simulink model "MOTORfault"  (R2018a)
settings: Solver=ode23tb  StartTime=0.0  StopTime=5  RelTol=1e-3  EnableMultiTasking=on
libraries: powerlib x1
settings Model: Creator=MAY  LastModifiedBy=MAY
settings DataIOCC: LimitDataPoints=on  SaveFormat=Array  SignalLoggingSaveFormat=ModelDataLogs  SignalLoggingName=sigsOut
settings DebuggingCC: SaveWithParameterizedLinksMsg=none  UnderspecifiedInitializationDetection=Classic  MergeDetectMultiDrivingBlocksExec=none  SignalResolutionControl=TryResolveAllWithWarning  MultiTaskDSMMsg=warning  MultiTaskCondExecSysMsg=none
settings HardwareCC: ProdBitPerPointer=32  ProdBitPerSizeT=32  ProdBitPerPtrDiffT=32  ProdLargestAtomicFloat=None  ProdIntDivRoundTo=Undefined  ProdEndianess=Unspecified  ProdWordSize=32  ProdHWDeviceType=32-bit Generic  TargetUnknown=on
settings ModelReferenceCC: PropagateSignalLabelsOutOfModel=off
settings GRTTargetCC: TargetLangStandard=C89/C90 (ANSI)  CombineOutputUpdateFcns=off  GRTInterface=on
settings ConfigComp: CovMetricSettings=dw  CovHtmlReporting=on  CovSaveCumulativeToWorkspaceVar=on  CovSaveSingleToWorkspaceVar=on  CovExternalEMLEnable=off

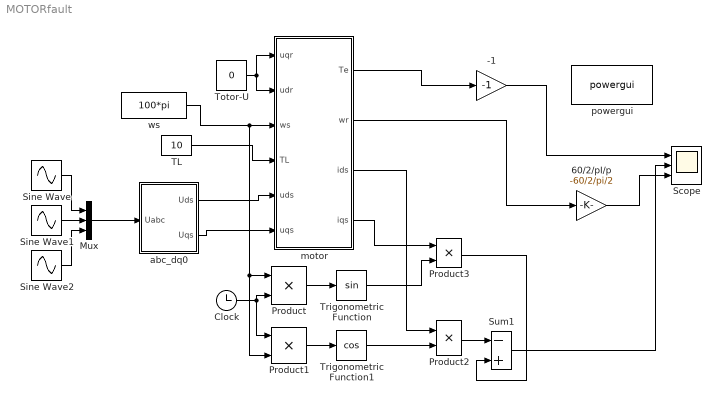
== system MOTORfault ==
  -1 : Gain  Gain=-1
  60/2/pI/p : Gain  Gain=-60/2/pi/2
  Clock : Clock
  Mux : Mux  Inputs=3
  Product{,1..3} (4 alike) : Product  SaturateOnIntegerOverflow=on  OutDataTypeStr=Inherit: Same as first input
  Scope : Scope  NumInputPorts=3
  Sine Wave : Sin  Amplitude=380  Frequency=2*pi*50  SampleTime=0
  Sine Wave1 : Sin  Amplitude=380  Frequency=2*pi*50  Phase=2*pi/3  SampleTime=0
  Sine Wave2 : Sin  Amplitude=380  Frequency=2*pi*50  Phase=-2*pi/3  SampleTime=0
  Sum1 : Sum  Inputs=-+  SaturateOnIntegerOverflow=on
  TL : Constant  Value=10
  Totor-U : Constant  Value=0
  Trigonometric Function : Trigonometry
  Trigonometric Function1 : Trigonometry  Operator=cos
  abc_dq0 : Subsystem
  motor : Subsystem
  powergui : powerlib/powergui  Priority=1  SimulationMode=Continuous  SampleTime=50e-6  frequency=60  Iterations=50  frequencyindice=60  Pbase=100e6  ErrMax=1e-4  UnitsV=kV  UnitsW=MW  buscounter=0  FunctionMessages=off  echomessages=off  EnableUseOfTLC=off  CurrentSourceSwitches=off  DisableSnubberDevices=off  DisableRonSwitches=off  DisableVfSwitches=off  DisplayEquations=off  SolverType=Tustin/Backward Euler (TBE)  Interpol=off  ExternalGateDelay=off  methode=off  Ts=100  x0status=blocks  SPID=on  SwTol=0  HookPort=off  RestoreLinks=warning  ResistiveCurrentMeasurement=off  Frange=[0:2:500]  Ylog=off  Xlog=on  ShowGrid=off  save=off  variable=ZData  structure=ScopeData  ZoomFFT=off  StartTime=4  cycles=50  DisplayStyle=3  fundamental=50  FreqAxis=off  MaxFrequency=120  frequencyindicesteady=1  RmsSteady=1  display=off
  ws : Constant  Value=100*pi
  wires:
  Mux/1 -> abc_dq0/1(Uabc)
  motor/4(iqs) -> Product3/1
  abc_dq0/1(Uds) -> motor/5(uds)
  abc_dq0/2(Uqs) -> motor/6(uqs)
  Totor-U/1 -> motor/1(uqr), motor/2(udr)
  Sine Wave1/1 -> Mux/2
  Sine Wave/1 -> Mux/1
  Sine Wave2/1 -> Mux/3
  motor/2(wr) -> 60/2/pI/p/1
  60/2/pI/p/1 -> Scope/3
  TL/1 -> motor/4(TL)
  motor/1(Te) -> -1/1
  -1/1 -> Scope/1
  ws/1 -> motor/3(ws), Product/1, Product1/2
  Trigonometric Function/1 -> Product3/2
  Product3/1 -> Sum1/2
  Product2/1 -> Sum1/1
  Product/1 -> Trigonometric Function/1
  Trigonometric Function1/1 -> Product2/2
  Product1/1 -> Trigonometric Function1/1
  motor/3(ids) -> Product2/1
  Sum1/1 -> Scope/2
  Clock/1 -> Product1/1, Product/2

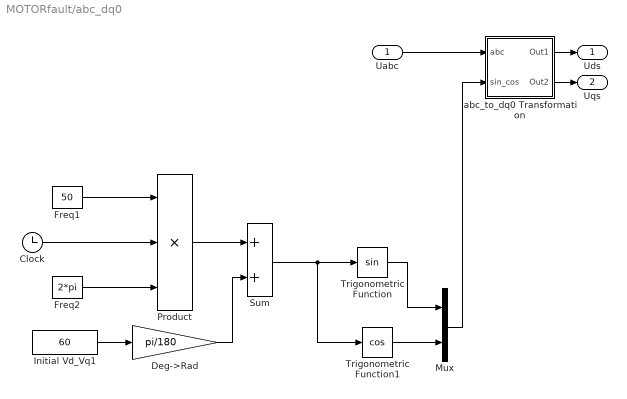
== system MOTORfault/abc_dq0 ==
  Uabc : Inport
  Clock : Clock
  Deg->Rad : Gain  Gain=pi/180  SaturateOnIntegerOverflow=on  OutDataTypeStr=Inherit: Same as input  ParamDataTypeStr=Inherit: Same as input
  Freq1 : Constant  Value=50
  Freq2 : Constant  Value=2*pi
  Initial Vd_Vq1 : Constant  Value=60
  Mux : Mux  Inputs=2
  Product : Product  Inputs=***  SaturateOnIntegerOverflow=on  InputSameDT=on  OutDataTypeStr=Inherit: Same as first input
  Sum : Sum  SaturateOnIntegerOverflow=on  InputSameDT=on  OutDataTypeStr=Inherit: Same as first input
  Trigonometric Function : Trigonometry
  Trigonometric Function1 : Trigonometry  Operator=cos
  abc_to_dq0 Transformation : Subsystem  mask(abc to dq0 Transformation){}
      mask help:
      | This block performs the  abc to dq0 transformation on a set of three-phase signals. It computes the direct axis Vd, quadratic axis Vq, and zero sequence V0 quantities in a two axis rotating reference frame according to the following transformation:
      |
      | Vd = 2/3*[Va*sin(wt)  + Vb*sin(wt-2pi/3)  +  Vc*sin(wt+2pi/3)]
      | Vq = 2/3*[Va*cos(wt) + Vb*cos(wt-2pi/3) + Vc*cos(wt+2pi/3)]
      | V0 = 1/3*[Va +  Vb  +  Vc ]
      |
      | where w=  rotation speed (rad/s) of the rotating frame.
      |
      | This transformation is commonly used in three-phase electric machine models where it is known as the Park transformation.
      mask Help: web(psbhelp);
  Uds : Outport
  Uqs : Outport  Port=2
  wires:
  Mux/1 -> abc_to_dq0 Transformation/2(sin_cos)
  Trigonometric Function1/1 -> Mux/2
  Trigonometric Function/1 -> Mux/1
  Sum/1 -> Trigonometric Function/1, Trigonometric Function1/1
  Product/1 -> Sum/1
  Initial Vd_Vq1/1 -> Deg->Rad/1
  Deg->Rad/1 -> Sum/2
  Freq1/1 -> Product/1
  Freq2/1 -> Product/3
  Clock/1 -> Product/2
  abc_to_dq0 Transformation/1(Out1) -> Uds/1
  abc_to_dq0 Transformation/2(Out2) -> Uqs/1
  Uabc/1 -> abc_to_dq0 Transformation/1(abc)

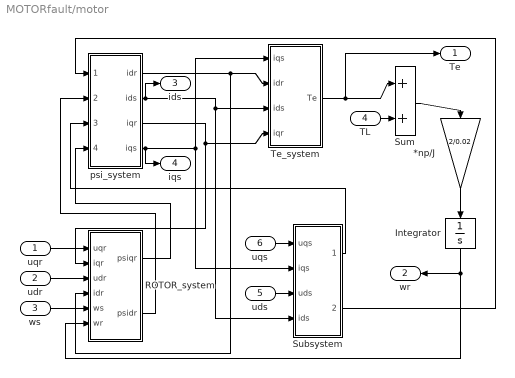
== system MOTORfault/motor ==
  uqr : Inport
  udr : Inport  Port=2
  ws : Inport  Port=3
  TL : Inport  Port=4
  uds : Inport  Port=5
  uqs : Inport  Port=6
  *np/J : Gain  Gain=2/0.02  SaturateOnIntegerOverflow=on  OutDataTypeStr=Inherit: Same as input  ParamDataTypeStr=Inherit: Same as input
  Integrator : Integrator
  ROTOR_system : Subsystem
  Subsystem : Subsystem
  Sum : Sum  SaturateOnIntegerOverflow=on
  Te_system : Subsystem
  psi_system : Subsystem
  Te : Outport
  wr : Outport  Port=2
  ids : Outport  Port=3
  iqs : Outport  Port=4
  wires:
  uqr/1 -> ROTOR_system/1(uqr)
  udr/1 -> ROTOR_system/3(udr)
  ws/1 -> ROTOR_system/5(ws)
  uds/1 -> Subsystem/3(uds)
  uqs/1 -> Subsystem/1(uqs)
  Integrator/1 -> ROTOR_system/6(wr), wr/1
  Sum/1 -> *np/J/1
  *np/J/1 -> Integrator/1
  Subsystem/1(psiqs) -> psi_system/3(ps1_qs)
  Subsystem/2(psids) -> psi_system/1(ps1_ds)
  ROTOR_system/2(psidr) -> psi_system/2(ps1_dr)
  ROTOR_system/1(psiqr) -> psi_system/4(ps1_qr)
  Te_system/1(Te) -> Sum/1, Te/1
  psi_system/4(iqs) -> Te_system/1(iqs), Subsystem/2(iqs), iqs/1
  psi_system/3(iqr) -> Te_system/4(iqr), ROTOR_system/2(iqr)
  psi_system/2(ids) -> Te_system/3(ids), Subsystem/4(ids), ids/1
  psi_system/1(idr) -> Te_system/2(idr), ROTOR_system/4(idr)
  TL/1 -> Sum/2

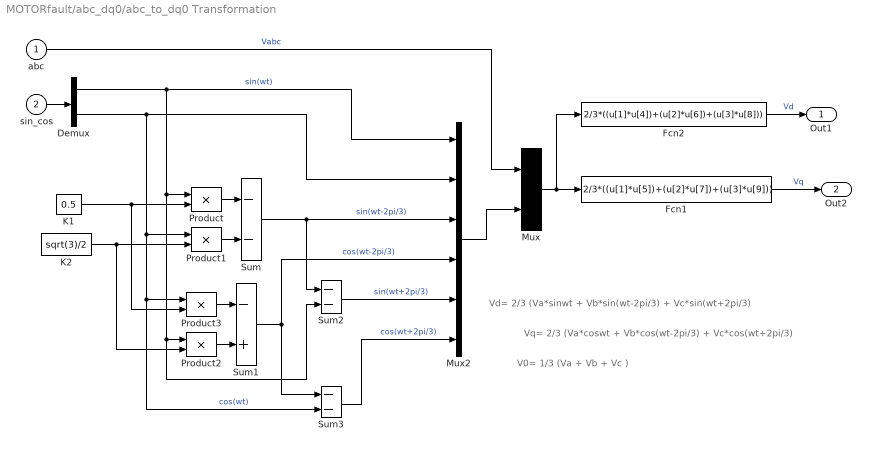
== system MOTORfault/abc_dq0/abc_to_dq0 Transformation ==
  note: V0= 1/3 (Va + Vb + Vc )
  note: Vd= 2/3 (Va*sinwt + Vb*sin(wt-2pi/3) + Vc*sin(wt+2pi/3)
  note: Vq= 2/3 (Va*coswt + Vb*cos(wt-2pi/3) + Vc*cos(wt+2pi/3)
  abc : Inport  PortDimensions=3
  sin_cos : Inport  Port=2  PortDimensions=2
  Demux : Demux  Outputs=2
  Fcn1 : Fcn  Expr=2/3*((u[1]*u[5])+(u[2]*u[7])+(u[3]*u[9]))
  Fcn2 : Fcn  Expr=2/3*((u[1]*u[4])+(u[2]*u[6])+(u[3]*u[8]))
  K1 : Constant  Value=0.5
  K2 : Constant  Value=sqrt(3)/2
  Mux : Mux  Inputs=2
  Mux2 : Mux  Inputs=6
  Product{,1..3} (4 alike) : Product  SaturateOnIntegerOverflow=on  InputSameDT=on  OutDataTypeStr=Inherit: Same as first input
  Sum : Sum  Inputs=--  SaturateOnIntegerOverflow=on  InputSameDT=on  OutDataTypeStr=Inherit: Same as first input
  Sum1 : Sum  Inputs=-+  SaturateOnIntegerOverflow=on  InputSameDT=on  OutDataTypeStr=Inherit: Same as first input
  Sum2 : Sum  Inputs=--  SaturateOnIntegerOverflow=on  InputSameDT=on  OutDataTypeStr=Inherit: Same as first input
  Sum3 : Sum  Inputs=--  SaturateOnIntegerOverflow=on  InputSameDT=on  OutDataTypeStr=Inherit: Same as first input
  Out1 : Outport
  Out2 : Outport  Port=2
  wires:
  Mux/1 -> Fcn1/1, Fcn2/1
  Sum1/1 -> Sum3/1, Mux2/4  "cos(wt-2pi/3)"
  Sum/1 -> Sum2/1, Mux2/3  "sin(wt-2pi/3)"
  K2/1 -> Product2/2, Product1/2
  K1/1 -> Product3/2, Product/2
  Sum2/1 -> Mux2/5  "sin(wt+2pi/3)"
  Sum3/1 -> Mux2/6  "cos(wt+2pi/3)"
  Product2/1 -> Sum1/2
  Product3/1 -> Sum1/1
  Product1/1 -> Sum/2
  Product/1 -> Sum/1
  Demux/1 -> Mux2/1, Sum2/2, Product2/1, Product/1  "sin(wt)"
  Demux/2 -> Mux2/2, Product1/1, Product3/1, Sum3/2  "cos(wt)"
  sin_cos/1 -> Demux/1
  Mux2/1 -> Mux/2
  abc/1 -> Mux/1  "Vabc"
  Fcn2/1 -> Out1/1  "Vd"
  Fcn1/1 -> Out2/1  "Vq"

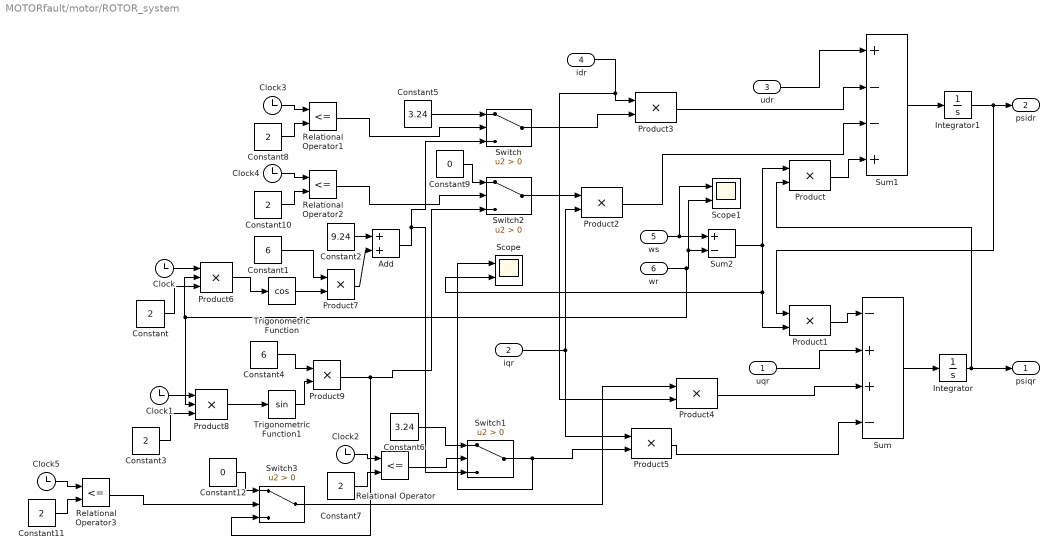
== system MOTORfault/motor/ROTOR_system ==
  uqr : Inport
  iqr : Inport  Port=2
  udr : Inport  Port=3
  idr : Inport  Port=4
  ws : Inport  Port=5
  wr : Inport  Port=6
  Add : Sum
  Clock{,1..5} (6 alike) : Clock
  Constant{,3,7..8,10..11} (6 alike) : Constant  Value=2
  Constant1 : Constant  Value=6
  Constant12 : Constant  Value=0
  Constant2 : Constant  Value=9.24
  Constant4 : Constant  Value=6
  Constant5 : Constant  Value=3.24
  Constant6 : Constant  Value=3.24
  Constant9 : Constant  Value=0
  Integrator : Integrator
  Integrator1 : Integrator
  Product{,1..5,7,9} (8 alike) : Product  SaturateOnIntegerOverflow=on  OutDataTypeStr=Inherit: Same as first input
  Product6 : Product  Inputs=3  SaturateOnIntegerOverflow=on  OutDataTypeStr=Inherit: Same as first input
  Product8 : Product  Inputs=3  SaturateOnIntegerOverflow=on  OutDataTypeStr=Inherit: Same as first input
  Relational Operator{,1..3} (4 alike) : RelationalOperator  Operator=<=  OutDataTypeStr=boolean  RndMeth=Simplest
  Scope : Scope  NumInputPorts=2
  Scope1 : Scope  NumInputPorts=2
  Sum : Sum  Inputs=-++-  SaturateOnIntegerOverflow=on
  Sum1 : Sum  Inputs=+--+  SaturateOnIntegerOverflow=on
  Sum2 : Sum  Inputs=+-  SaturateOnIntegerOverflow=on
  Switch{,1..3} (4 alike) : Switch  Criteria=u2 > Threshold
  Trigonometric Function : Trigonometry  Operator=cos
  Trigonometric Function1 : Trigonometry
  psiqr : Outport
  psidr : Outport  Port=2
  wires:
  Sum/1 -> Integrator/1
  Integrator/1 -> psiqr/1, Product/2
  uqr/1 -> Sum/2
  Sum1/1 -> Integrator1/1
  Integrator1/1 -> psidr/1, Product1/1
  udr/1 -> Sum1/1
  Product/1 -> Sum1/4
  Product1/1 -> Sum/1
  wr/1 -> Product8/2, Product6/2, Scope1/2, Sum2/2
  ws/1 -> Scope1/1, Sum2/1
  idr/1 -> Product4/2, Product3/1
  Product3/1 -> Sum1/2
  Product2/1 -> Sum1/3
  Product4/1 -> Sum/3
  Product5/1 -> Sum/4
  iqr/1 -> Product5/1, Product2/2
  Add/1 -> Switch/3, Switch1/3
  Clock/1 -> Product6/1
  Product6/1 -> Trigonometric Function/1
  Trigonometric Function/1 -> Product7/2
  Constant/1 -> Product6/3
  Constant1/1 -> Product7/1
  Product7/1 -> Add/2
  Constant2/1 -> Add/1
  Constant3/1 -> Product8/3
  Clock1/1 -> Product8/1
  Trigonometric Function1/1 -> Product9/2
  Sum2/1 -> Scope/2, Product1/2, Product/1
  Product8/1 -> Trigonometric Function1/1
  Constant4/1 -> Product9/1
  Switch/1 -> Product3/2
  Constant5/1 -> Switch/1
  Switch1/1 -> Scope/1, Product5/2
  Constant6/1 -> Switch1/1
  Clock2/1 -> Relational Operator/1
  Constant7/1 -> Relational Operator/2
  Relational Operator/1 -> Switch1/2
  Relational Operator1/1 -> Switch/2
  Clock3/1 -> Relational Operator1/1
  Constant8/1 -> Relational Operator1/2
  Product9/1 -> Switch3/3, Switch2/3
  Clock4/1 -> Relational Operator2/1
  Constant10/1 -> Relational Operator2/2
  Relational Operator2/1 -> Switch2/2
  Switch2/1 -> Product2/1
  Constant9/1 -> Switch2/1
  Constant11/1 -> Relational Operator3/2
  Constant12/1 -> Switch3/1
  Relational Operator3/1 -> Switch3/2
  Clock5/1 -> Relational Operator3/1
  Switch3/1 -> Product4/1

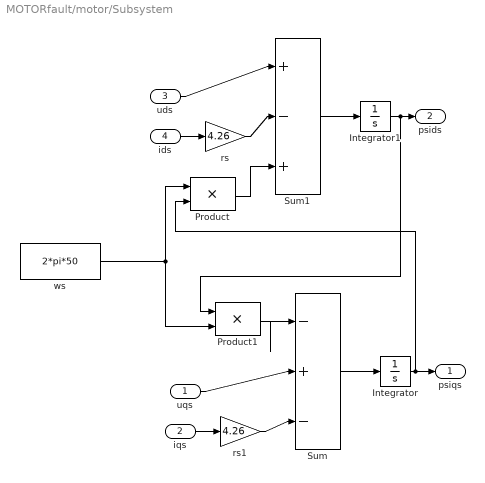
== system MOTORfault/motor/Subsystem ==
  uqs : Inport
  iqs : Inport  Port=2
  uds : Inport  Port=3
  ids : Inport  Port=4
  Integrator : Integrator
  Integrator1 : Integrator
  Product : Product  SaturateOnIntegerOverflow=on  OutDataTypeStr=Inherit: Same as first input
  Product1 : Product  SaturateOnIntegerOverflow=on  OutDataTypeStr=Inherit: Same as first input
  Sum : Sum  Inputs=|-+-  SaturateOnIntegerOverflow=on
  Sum1 : Sum  Inputs=|+-+  SaturateOnIntegerOverflow=on
  rs : Gain  Gain=4.26  SaturateOnIntegerOverflow=on  OutDataTypeStr=Inherit: Same as input  ParamDataTypeStr=Inherit: Same as input
  rs1 : Gain  Gain=4.26  SaturateOnIntegerOverflow=on  OutDataTypeStr=Inherit: Same as input  ParamDataTypeStr=Inherit: Same as input
  ws : Constant  Value=2*pi*50
  psiqs : Outport
  psids : Outport  Port=2
  wires:
  rs1/1 -> Sum/3
  Sum/1 -> Integrator/1
  Integrator/1 -> psiqs/1, Product/2
  uqs/1 -> Sum/2
  iqs/1 -> rs1/1
  rs/1 -> Sum1/2
  Sum1/1 -> Integrator1/1
  Integrator1/1 -> psids/1, Product1/1
  uds/1 -> Sum1/1
  ids/1 -> rs/1
  ws/1 -> Product/1, Product1/2
  Product1/1 -> Sum/1
  Product/1 -> Sum1/3

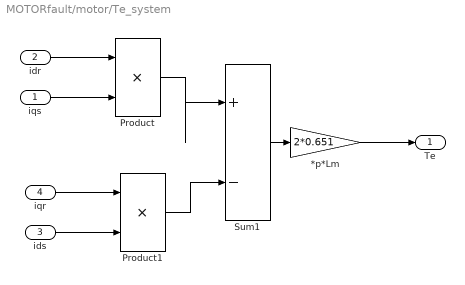
== system MOTORfault/motor/Te_system ==
  iqs : Inport
  idr : Inport  Port=2
  ids : Inport  Port=3
  iqr : Inport  Port=4
  *p*Lm : Gain  Gain=2*0.651  SaturateOnIntegerOverflow=on  OutDataTypeStr=Inherit: Same as input  ParamDataTypeStr=Inherit: Same as input
  Product : Product  SaturateOnIntegerOverflow=on  OutDataTypeStr=Inherit: Same as first input
  Product1 : Product  SaturateOnIntegerOverflow=on  OutDataTypeStr=Inherit: Same as first input
  Sum1 : Sum  Inputs=|+-  SaturateOnIntegerOverflow=on
  Te : Outport
  wires:
  idr/1 -> Product/1
  iqs/1 -> Product/2
  iqr/1 -> Product1/1
  ids/1 -> Product1/2
  Product/1 -> Sum1/1
  Product1/1 -> Sum1/2
  Sum1/1 -> *p*Lm/1
  *p*Lm/1 -> Te/1

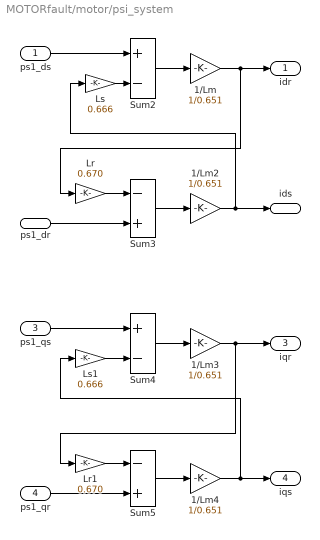
== system MOTORfault/motor/psi_system ==
  ps1_ds : Inport
  ps1_dr : Inport  Port=2
  ps1_qs : Inport  Port=3
  ps1_qr : Inport  Port=4
  1/Lm{,2..4} (4 alike) : Gain  Gain=1/0.651  SaturateOnIntegerOverflow=on  OutDataTypeStr=Inherit: Same as input  ParamDataTypeStr=Inherit: Same as input
  Lr : Gain  Gain=0.670  SaturateOnIntegerOverflow=on  OutDataTypeStr=Inherit: Same as input  ParamDataTypeStr=Inherit: Same as input
  Lr1 : Gain  Gain=0.670  SaturateOnIntegerOverflow=on  OutDataTypeStr=Inherit: Same as input  ParamDataTypeStr=Inherit: Same as input
  Ls : Gain  Gain=0.666  SaturateOnIntegerOverflow=on  OutDataTypeStr=Inherit: Same as input  ParamDataTypeStr=Inherit: Same as input
  Ls1 : Gain  Gain=0.666  SaturateOnIntegerOverflow=on  OutDataTypeStr=Inherit: Same as input  ParamDataTypeStr=Inherit: Same as input
  Sum2 : Sum  Inputs=+-  SaturateOnIntegerOverflow=on
  Sum3 : Sum  Inputs=-+  SaturateOnIntegerOverflow=on
  Sum4 : Sum  Inputs=+-  SaturateOnIntegerOverflow=on
  Sum5 : Sum  Inputs=-+  SaturateOnIntegerOverflow=on
  idr : Outport
  ids : Outport  Port=2
  iqr : Outport  Port=3
  iqs : Outport  Port=4
  wires:
  ps1_ds/1 -> Sum2/1
  Sum2/1 -> 1/Lm/1
  1/Lm/1 -> idr/1, Lr/1
  1/Lm2/1 -> ids/1, Ls/1
  ps1_qs/1 -> Sum4/1
  Sum4/1 -> 1/Lm3/1
  1/Lm3/1 -> iqr/1, Lr1/1
  Sum5/1 -> 1/Lm4/1
  1/Lm4/1 -> iqs/1, Ls1/1
  ps1_dr/1 -> Sum3/2
  Sum3/1 -> 1/Lm2/1
  Lr/1 -> Sum3/1
  ps1_qr/1 -> Sum5/2
  Lr1/1 -> Sum5/1
  Ls/1 -> Sum2/2
  Ls1/1 -> Sum4/2
